simulink model "Velo_BF_test"  (R2018a)
settings: Solver=ode15s  StartTime=0.0  StopTime=10  FixedStep=0.00001  RelTol=1e-5  AbsTol=1e-3
undefined symbols (not defined in the file): g, Jr, Jv, Kd_v, Ki_v, Kp_v, Lr, Lv, Mr, Mv
libraries: cstblocks x1
settings Model: Creator=chsira  LastModifiedBy=charl
settings SolverCC: SolverResetMethod=Robust
settings DebuggingCC: LibraryContextMissingDiagnostic=warning
settings ModelReferenceCC: ModelReferenceMinAlgLoopOccurrences=on
settings SFSimCC: SimUseLocalCustomCode=on
settings RTWCC: RTWUseLocalCustomCode=on

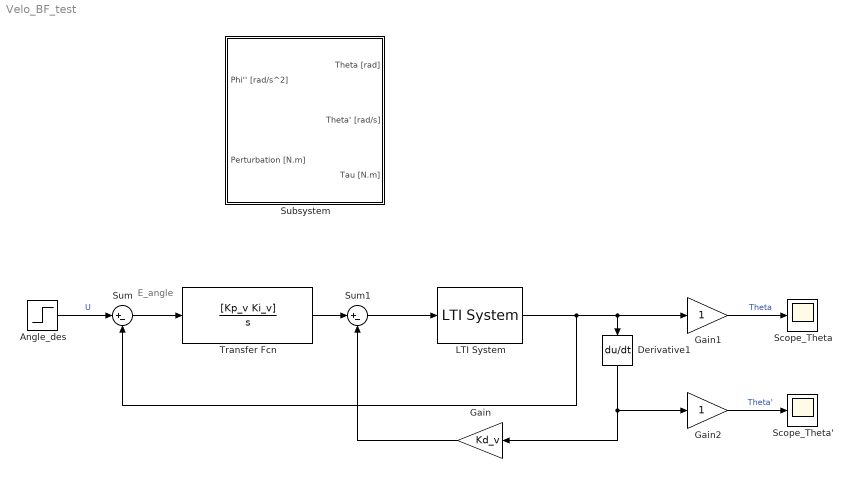
== system Velo_BF_test ==
  note: E_angle
  "Angle_des " : Step  Time=0  SampleTime=0
  Derivative1 : Derivative
  Gain : Gain  Gain=Kd_v
  Gain1 : Gain
  Gain2 : Gain
  LTI System : cstblocks/LTI System  sys=G_a  IC=[]
  Scope_Theta : Scope
  Scope_Theta' : Scope
  Subsystem : Subsystem  mask{InitialCondition=0*pi/180}
      mask prompts: InitialCondition "Angle initial"
      mask TypeOptions InitialCondition: Integrator1/InitialCondition
  Sum : Sum  Inputs=|+-
  Sum1 : Sum  Inputs=|+-
  Transfer Fcn : TransferFcn  Numerator=[Kp_v Ki_v]  Denominator=[1 0]
  wires:
  LTI System/1 -> Gain1/1, Derivative1/1, Sum/2
  "Angle_des "/1 -> Sum/1  "U"
  Sum/1 -> Transfer Fcn/1
  Gain1/1 -> Scope_Theta/1  "Theta"
  Gain2/1 -> Scope_Theta'/1  "Theta'"
  Derivative1/1 -> Gain/1, Gain2/1
  Transfer Fcn/1 -> Sum1/1
  Sum1/1 -> LTI System/1
  Gain/1 -> Sum1/2

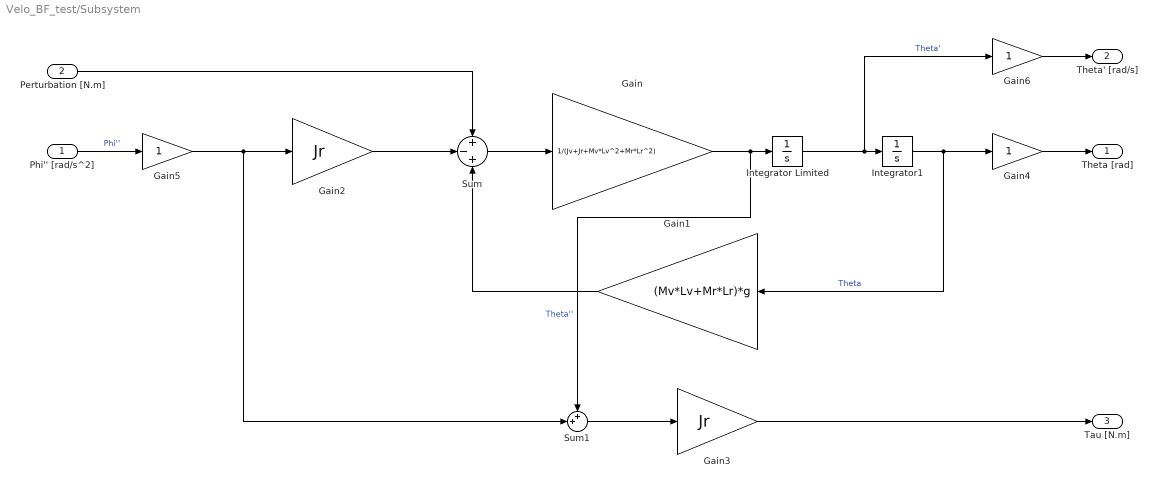
== system Velo_BF_test/Subsystem ==
  Phi'' [rad/s^2] : Inport  OutDataTypeStr=double  PortDimensions=1  SampleTime=0
  Perturbation [N.m] : Inport  Port=2  OutDataTypeStr=double  PortDimensions=1  SampleTime=0
  Gain : Gain  Gain=1/(Jv+Jr+Mv*Lv^2+Mr*Lr^2)
  Gain1 : Gain  Gain=(Mv*Lv+Mr*Lr)*g
  Gain2 : Gain  Gain=Jr
  Gain3 : Gain  Gain=Jr
  Gain4 : Gain
  Gain5 : Gain
  Gain6 : Gain
  Integrator Limited : Integrator  InitialCondition=0.00001  LimitOutput=on  UpperSaturationLimit=10000000  LowerSaturationLimit=-10000000
  Integrator1 : Integrator  InitialCondition=InitialCondition  mask{InitialCondition=InitialCondition}
      mask prompts: InitialCondition "Angle initial"
      mask TypeOptions InitialCondition: InitialCondition
  Sum : Sum  Inputs=+-+
  Sum1 : Sum  Inputs=++|
  Theta [rad] : Outport  OutDataTypeStr=double  PortDimensions=1  SampleTime=0
  Theta' [rad/s] : Outport  Port=2  OutDataTypeStr=double  PortDimensions=1  SampleTime=0
  "Tau [N.m] " : Outport  Port=3  OutDataTypeStr=double  PortDimensions=1  SampleTime=0
  wires:
  Gain5/1 -> Gain2/1, Sum1/2
  Integrator Limited/1 -> Integrator1/1, Gain6/1  "Theta'"
  Gain2/1 -> Sum/2
  Gain4/1 -> Theta [rad]/1
  Gain1/1 -> Sum/3
  Gain6/1 -> Theta' [rad/s]/1
  Sum/1 -> Gain/1
  Gain/1 -> Integrator Limited/1, Sum1/1  "Theta''"
  Integrator1/1 -> Gain1/1, Gain4/1  "Theta"
  Perturbation [N.m]/1 -> Sum/1
  Sum1/1 -> Gain3/1
  Gain3/1 -> "Tau [N.m] "/1
  Phi'' [rad/s^2]/1 -> Gain5/1  "Phi''"
